simulink model "HVModAL_Fahrzeugmodell"  (R2015b)
settings: Solver=ode1  StartTime=0  StopTime=drp.driving_cycle.tstop  FixedStep=sim_params.Ts  RelTol=1e-5
PreLoadFcn:
  | % Add paths
  | addpath data
  | addpath(genpath('library'))
StartFcn:
  | Simulation.StartTime = tic;
StopFcn:
  | Simulation.DurationTime = toc(Simulation.StartTime);
undefined symbols (not defined in the file or in its folder): Batteries, BMS, BMS_Bat_, C_Nenn_DCDC1, C_Nenn_DCDC2, d2d, DC, DCDC_Converter_efficiency, DcDc_Converters, Dcl, drp, drv, elm, gen, gin, Hdc, hdc, HV, hvb, Hvb, ice, ldc, lib_dcl, lib_hdc, lib_hvb, lib_veh, Link, lossestable, mask_LUT_OCV, mask_LUT_OCV_SOC, mask_LUT_OCV_Temperature, mask_LUT_R, mask_LUT_Rs, mask_LUT_Rs_SOC, mask_LUT_Rs_Temperature, sim_params, speedvec, torquevec, tri, veh, Veh, Vehicle_Chassis
libraries: simulink x29, lib_tri_modules x7, lib_hdc_module x5, lib_gearbox x4, lib_hvb_battery_pack x3, cstblocks x3, PowerLimitBlock x2, MultiCellLibrary x2, lib_aux x1, lib_drv x1, lib_gen x1, lib_elm x1
(part 1 of 7)
settings Model: Creator=abu  LastModifiedBy=hangyang
settings SolverCC: AutoInsertRateTranBlk=on
settings DataIOCC: SaveFormat=Array  SignalLoggingSaveFormat=ModelDataLogs
settings OptimizationCC: DefaultParameterBehavior=Inlined
settings DebuggingCC: ReadBeforeWriteMsg=DisableAll  WriteAfterWriteMsg=DisableAll  WriteAfterReadMsg=DisableAll  CheckSSInitialOutputMsg=off  UnderspecifiedInitializationDetection=Classic  MergeDetectMultiDrivingBlocksExec=none  SolverPrmCheckMsg=warning  MultiTaskDSMMsg=none  MultiTaskCondExecSysMsg=none  UnconnectedInputMsg=none  UnconnectedOutputMsg=none  UnconnectedLineMsg=none  StateNameClashWarn=warning
settings HardwareCC: ProdBitPerPointer=32  ProdLargestAtomicFloat=None  ProdIntDivRoundTo=Undefined  ProdEndianess=Unspecified  ProdWordSize=32  ProdHWDeviceType=32-bit Generic
settings ModelReferenceCC: UpdateModelReferenceTargets=IfOutOfDate
settings SFSimCC: SFSimEcho=off
settings GRTTargetCC: GeneratePreprocessorConditionals=Disable all
settings ConfigComp: CovModelRefEnable=Off  CovSFcnEnable=off

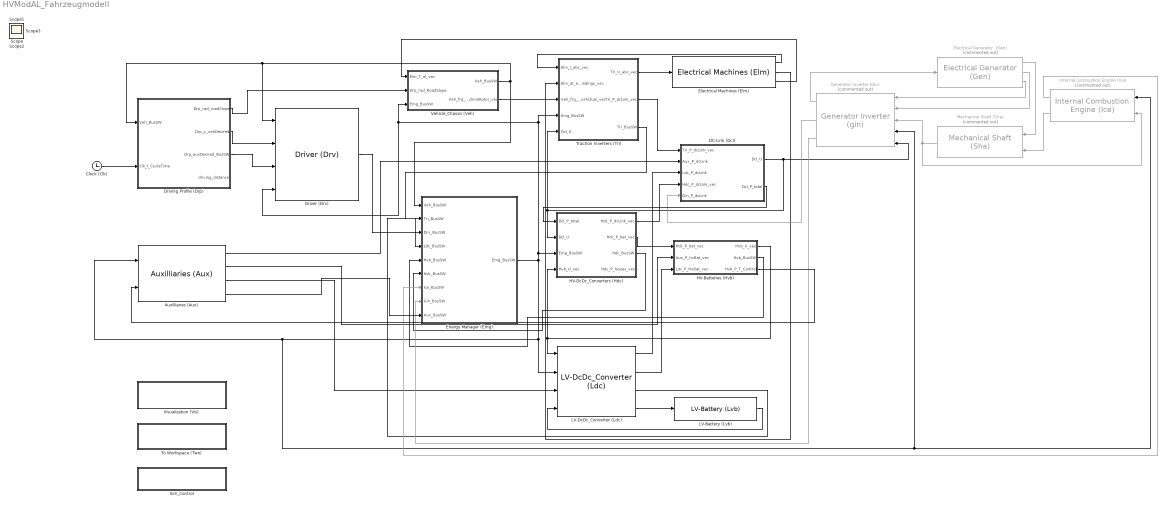
== system HVModAL_Fahrzeugmodell ==
  Auxilliaries (Aux) : lib_aux/Auxilliaries (Aux)
  Clock (Clk) : Clock
  DC-Link (Dcl) : Subsystem  AncestorBlock=lib_dcl/DC-Link (Dcl)
  Driver (Drv) : lib_drv/Driver (Drv)
  Driving Profile (Drp) : Subsystem  AncestorBlock=lib_drp/Driving Profile (Drp)
  Electrical Generator  (Gen) : lib_gen/Electrical Generator  (Gen)  Commented=on
  Electrical Machines (Elm) : lib_elm/Electrical Machines (Elm)
  Energy Manager (Emg) : Subsystem  AncestorBlock=lib_emg/Energy Manager (Emg)
  Generator Inverter (Gin) : lib_gin/Generator Inverter (gin)  Commented=on
  HV-Batteries (Hvb) : Subsystem  AncestorBlock=lib_hvb/HV-Batteries (Hvb)
  HV-DcDc_Converters (Hdc) : Subsystem  AncestorBlock=lib_hdc/HV-DcDc_Converters (Hdc)
  Internal Combustion Engine (Ice) : lib_ice/Internal Combustion Engine (Ice)  Commented=on
  LV-Battery (Lvb) : lib_lvb/LV-Battery (Lvb)
  LV-DcDc_Converter (Ldc) : lib_ldc/LV-DcDc_Converter (Ldc)
  Mechanical Shaft (Sha) : lib_Sha/Mechanical Shaft (Sha)  Commented=on
  Sim_Control : Subsystem
  To Workspace (Two) : Subsystem
  Traction Inverters (Tri) : Subsystem  AncestorBlock=lib_tri/Traction Inverters (Tri)
  Vehicle_Chassis (Veh) : Subsystem  AncestorBlock=lib_veh/Vehicle_Chassis (Veh)
  Visualization (Vis) : Subsystem
  Scope{,1..3} (4 alike) : Scope
  wires:
  Clock (Clk)/1 -> Driving Profile (Drp)/2(Clk_t_CycleTime)
  HV-Batteries (Hvb)/1(Hvb_U_vec) -> LV-DcDc_Converter (Ldc)/1, HV-DcDc_Converters (Hdc)/4(Hvb_U_vec)
  Vehicle_Chassis (Veh)/1(Veh_BusSW) -> Energy Manager (Emg)/1(Veh_BusSW), Driver (Drv)/1, Driving Profile (Drp)/1(Veh_BusSW)
  LV-DcDc_Converter (Ldc)/2 -> HV-Batteries (Hvb)/3(Ldc_P_HvBat_vec)
  Traction Inverters (Tri)/1(Tri_U_abc_vec) -> Electrical Machines (Elm)/1
  LV-DcDc_Converter (Ldc)/4 -> LV-Battery (Lvb)/1
  LV-Battery (Lvb)/1 -> LV-DcDc_Converter (Ldc)/4
  Driving Profile (Drp)/1(Drp_rad_roadSlope) -> Vehicle_Chassis (Veh)/2(Drp_rad_RoadSlope)
  Traction Inverters (Tri)/2(Tri_P_dcLink_vec) -> DC-Link (Dcl)/1(Tri_P_dcLink_vec)
  HV-DcDc_Converters (Hdc)/1(Hdc_P_dcLink_vec) -> DC-Link (Dcl)/4(Hdc_P_dcLink_vec)
  Auxilliaries (Aux)/3 -> LV-DcDc_Converter (Ldc)/3
  LV-DcDc_Converter (Ldc)/1 -> DC-Link (Dcl)/3(Ldc_P_dcLink)
  Energy Manager (Emg)/1(Emg_BusSW) -> Vehicle_Chassis (Veh)/3(Emg_BusSW), Driver (Drv)/4, Traction Inverters (Tri)/4(Emg_BusSW), HV-DcDc_Converters (Hdc)/3(Emg_BusSW), Internal Combustion Engine (Ice)/1, Generator Inverter (Gin)/4, Auxilliaries (Aux)/1, LV-DcDc_Converter (Ldc)/2
  DC-Link (Dcl)/1(Dcl_U) -> Traction Inverters (Tri)/5(Dcl_U), HV-DcDc_Converters (Hdc)/2(Dcl_U), Generator Inverter (Gin)/5
  Auxilliaries (Aux)/1 -> DC-Link (Dcl)/2(Aux_P_dcLink)
  HV-DcDc_Converters (Hdc)/2(Hdc_P_bat_vec) -> HV-Batteries (Hvb)/1(Hdc_P_bat_vec)
  Auxilliaries (Aux)/2 -> HV-Batteries (Hvb)/2(Aux_P_hvBat_vec)
  Vehicle_Chassis (Veh)/2(Veh_frq_machineRotor_vec) -> Traction Inverters (Tri)/3(Veh_frq_RotorActual_vec)
  Driver (Drv)/1 -> Energy Manager (Emg)/3("Drv_BusSW ")
  LV-DcDc_Converter (Ldc)/3 -> Energy Manager (Emg)/4(Ldc_BusSW)
  HV-DcDc_Converters (Hdc)/3(Hdc_BusSW) -> Energy Manager (Emg)/6(Hdc_BusSW)
  HV-Batteries (Hvb)/2(Hvb_BusSW) -> Energy Manager (Emg)/5(Hvb_BusSW)
  Traction Inverters (Tri)/3("Tri_BusSW ") -> Energy Manager (Emg)/2(Tri_BusSW)
  Electrical Machines (Elm)/1 -> Traction Inverters (Tri)/1(Elm_I_abc_vec)
  Electrical Machines (Elm)/2 -> Traction Inverters (Tri)/2(Elm_at_endWindings_vec)
  Generator Inverter (Gin)/2 -> DC-Link (Dcl)/5(Gin_P_dcLink)
  Generator Inverter (Gin)/1 -> Electrical Generator  (Gen)/1
  Electrical Generator  (Gen)/3 -> Generator Inverter (Gin)/1
  Electrical Generator  (Gen)/2 -> Generator Inverter (Gin)/2
  Mechanical Shaft (Sha)/1 -> Internal Combustion Engine (Ice)/2, Generator Inverter (Gin)/3
  Electrical Generator  (Gen)/1 -> Mechanical Shaft (Sha)/1
  Internal Combustion Engine (Ice)/2 -> Mechanical Shaft (Sha)/2
  Internal Combustion Engine (Ice)/1 -> Energy Manager (Emg)/7(Ice_BusSW)
  Generator Inverter (Gin)/3 -> Energy Manager (Emg)/8(Gin_BusSW)
  DC-Link (Dcl)/2(Dcl_P_total) -> HV-DcDc_Converters (Hdc)/1(Dcl_P_total)
  Electrical Machines (Elm)/3 -> Vehicle_Chassis (Veh)/1(Elm_T_el_vec)
  Driving Profile (Drp)/2(Drp_v_vehDesired) -> Driver (Drv)/2
  Driving Profile (Drp)/3(Drp_auxDesired_BusSW) -> Driver (Drv)/3
  Auxilliaries (Aux)/4 -> Energy Manager (Emg)/9("Aux_BusSW ")
  HV-Batteries (Hvb)/3(Hvb_P_T_Control) -> Auxilliaries (Aux)/2

== system HVModAL_Fahrzeugmodell/DC-Link (Dcl) ==
  note: edited by Jan: if this signal is cut, we don't have a direct algebraic loop
  Tri_P_dcLink_vec : Inport
  Aux_P_dcLink : Inport  Port=2
  Ldc_P_dcLink : Inport  Port=3
  Hdc_P_dcLink_vec : Inport  Port=4
  Gin_P_dcLink : Inport  Port=5
  Add : Sum  Inputs=+-
  Bus Creator : BusCreator  Inputs=4
  Dcl Voltage Calculation : Subsystem
  Delay : Delay  DelayLength=1  InitialCondition=0
  Gain : Gain  Gain=0
  Model Info : simulink/Model-Wide Utilities/Model Info  Frame=on  DisplayStringWithTags=|  HorizontalTextAlignment=Center  LeftAlignmentValue=0.5  SourceBlockDiagram=HVModAL_Fahrzeugmodell  TagMaxNumber=20
      | Responsibility
      | ISEA
      | 
      | Model Version: %<ModelVersion>
      | Last modified: %<LastModificationDate>
  Subtract1 : Sum  Inputs=+++++
  Sum of Elements : Sum  Inputs=+  SaturateOnIntegerOverflow=on
  Sum of Elements1 : Sum  Inputs=+  CollapseDim=2  SaturateOnIntegerOverflow=on
  Dcl_U : Outport
  Dcl_P_total : Outport  Port=2
  tag scope: Dcl_BusPB_toworkspace=global
  wires:
  Hdc_P_dcLink_vec/1 -> Sum of Elements/1
  Gin_P_dcLink/1 -> Gain/1
  Ldc_P_dcLink/1 -> Subtract1/4
  Sum of Elements/1 -> Delay/1
  Subtract1/1 -> Dcl Voltage Calculation/1(P), Bus Creator/3, Add/1  "Dcl_P_totalwoHdcPdcLink"
  Add/1 -> Dcl_P_total/1, Bus Creator/2  "Dcl_P_total"
  Aux_P_dcLink/1 -> Subtract1/3
  Gain/1 -> Subtract1/1
  Dcl Voltage Calculation/1(Dcl_U) -> Bus Creator/1, Dcl_U/1  "Dcl_U"
  Tri_P_dcLink_vec/1 -> Sum of Elements1/1
  Sum of Elements1/1 -> Subtract1/2
  Bus Creator/1 -> [Dcl_BusPB_toworkspace]
  Delay/1 -> Bus Creator/4  "Hdc_P_dcLink"

== system HVModAL_Fahrzeugmodell/Driving Profile (Drp) ==
  Veh_BusSW : Inport
  Clk_t_CycleTime : Inport  Port=2
  Bus Creator : BusCreator  Inputs=4
  Bus Creator1 : BusCreator  Inputs=3
  Load{1..4} (4 alike) : Constant  Value=0
  Model Info : simulink/Model-Wide Utilities/Model Info  Frame=on  DisplayStringWithTags=|  HorizontalTextAlignment=Center  LeftAlignmentValue=0.5  SourceBlockDiagram=HVModAL_Fahrzeugmodell  TagMaxNumber=20
      | Responsibility
      | ISEA
      | 
      | Model Version: %<ModelVersion>
      | Last modified: %<LastModificationDate>
  Slope Lookup : Lookup_n-D  NumberOfTableDimensions=1  BreakpointsForDimension1=drp.driving_cycle.slope(:,1)  Table=drp.driving_cycle.slope(:,2)  InternalRulePriority=Speed  RndMeth=Simplest  InputSameDT=on
  Speed Lookup : Lookup_n-D  NumberOfTableDimensions=1  BreakpointsForDimension1=drp.driving_cycle.speed(:,1)  Table=drp.driving_cycle.speed(:,2)  InternalRulePriority=Speed  RndMeth=Simplest  InputSameDT=on
  Terminator : Terminator
  drp_driving_distance[Km] : Constant  Value=500
  "km/h -> m/s" : Gain  Gain=1/3.6
  Drp_rad_roadSlope : Outport
  Drp_v_vehDesired : Outport  Port=2
  Drp_auxDesired_BusSW : Outport  Port=3
  "driving_distance " : Outport  Port=4
  tag scope: Drp_SWBus_toworkspace=global
  wires:
  "km/h -> m/s"/1 -> Bus Creator1/1, Drp_v_vehDesired/1  "Drp_v_vehDesired"
  Veh_BusSW/1 -> Terminator/1
  Clk_t_CycleTime/1 -> Slope Lookup/1, Speed Lookup/1
  Slope Lookup/1 -> Bus Creator1/2, Drp_rad_roadSlope/1  "Drp_rad_roadSlope"
  Bus Creator/1 -> Bus Creator1/3, Drp_auxDesired_BusSW/1  "Drp_auxDesired_BusSW"
  Load4/1 -> Bus Creator/4
  Load3/1 -> Bus Creator/3
  Load2/1 -> Bus Creator/2
  Load1/1 -> Bus Creator/1
  Bus Creator1/1 -> [Drp_SWBus_toworkspace]
  Speed Lookup/1 -> "km/h -> m/s"/1
  drp_driving_distance[Km]/1 -> "driving_distance "/1

== system HVModAL_Fahrzeugmodell/Energy Manager (Emg) ==
  note: Emg_battery_control_case
  note: Attention: SOC equalization strategy forced (27.9.16, JaB)
  Veh_BusSW : Inport
  Tri_BusSW : Inport  Port=2
  "Drv_BusSW " : Inport  Port=3
  Ldc_BusSW : Inport  Port=4
  Hvb_BusSW : Inport  Port=5
  Hdc_BusSW : Inport  Port=6
  Ice_BusSW : Inport  Port=7
  Gin_BusSW : Inport  Port=8
  "Aux_BusSW " : Inport  Port=9
  Aux Control : Subsystem
  Battery Control : Subsystem
  Battery Control1 : Subsystem  Commented=through
      mask help: Simulink:masks:GenSFuncDesc_MD
      mask Help: eval('feval(''rtwprivate'',''rtwhelpview'',''rtw_sfcn_block'')');
  Bus Creator : BusCreator  Inputs=13
  Emg_P_lvDemand : Constant  Value=0
  Emg_P_lvDemand1 : Constant  Value=0
  Emg_U_dcLinkDemand : Constant  Value=veh.topology.Dcl_U
  Model Info : simulink/Model-Wide Utilities/Model Info  Frame=on  DisplayStringWithTags=|  HorizontalTextAlignment=Center  LeftAlignmentValue=0.5  SourceBlockDiagram=HVModAL_Fahrzeugmodell  TagMaxNumber=20
      | Responsibility
      | ISEA
      | 
      | Model Version: %<ModelVersion>
      | Last modified: %<LastModificationDate>
  Mux : Mux  Inputs=3
  Range Extender Control : Subsystem
  Terminator2 : Terminator
  "Torque Control motor (1 elm, 1 tri, 2 hdc, 2 bat)" : Torque_Control/Torque Control motor (1 elm, 1 tri, 2 hdc, 2 bat)
  at_Ambient : Constant  Value=25
  Emg_BusSW : Outport
  tag scope: EMG_BusSW_ToLogging=global, EMG_BusSW_ToWorkspace=global
  wires:
  Emg_P_lvDemand/1 -> Mux/3  "Emg_P_lvDemand"
  Emg_U_dcLinkDemand/1 -> Bus Creator/6  "Emg_U_dcLinkDemand"
  Bus Creator/1 -> Emg_BusSW/1, [EMG_BusSW_ToWorkspace], [EMG_BusSW_ToLogging]
  Tri_BusSW/1 -> "Torque Control motor (1 elm, 1 tri, 2 hdc, 2 bat)"/5, Aux Control/4(Tri_BusSW), Battery Control/3(Tri_BusSW)
  Ldc_BusSW/1 -> Terminator2/1
  Hdc_BusSW/1 -> "Torque Control motor (1 elm, 1 tri, 2 hdc, 2 bat)"/4
  Ice_BusSW/1 -> Range Extender Control/1(Ice_BusSW)
  Gin_BusSW/1 -> Range Extender Control/2(Gin_BusSW)
  Hvb_BusSW/1 -> Battery Control/1(Hvb_BusSW), "Torque Control motor (1 elm, 1 tri, 2 hdc, 2 bat)"/6
  Range Extender Control/1(Emg_fac_GenDeman) -> Bus Creator/9  "Emg_fac_GenDeman"
  "Torque Control motor (1 elm, 1 tri, 2 hdc, 2 bat)"/1 -> Bus Creator/1  "Emg_T_elDemand_vec"
  "Drv_BusSW "/1 -> "Torque Control motor (1 elm, 1 tri, 2 hdc, 2 bat)"/2
  "Torque Control motor (1 elm, 1 tri, 2 hdc, 2 bat)"/2 -> Bus Creator/2  "Emg_T_mechDemand"
  Battery Control/1(Emg_fac_powerDistribution_vec) -> Bus Creator/5  "Emg_fac_powerDistribution_vec"
  Aux Control/1(Emg_auxControl_BusSW) -> Bus Creator/8
  Veh_BusSW/1 -> Battery Control/2(Veh_BusSW), "Torque Control motor (1 elm, 1 tri, 2 hdc, 2 bat)"/3
  Mux/1 -> Bus Creator/7  "Emg_P_lvdemand"
  Emg_P_lvDemand1/1 -> Mux/2, Mux/1
  at_Ambient/1 -> Bus Creator/10  "Emg_at_Ambient"
  "Torque Control motor (1 elm, 1 tri, 2 hdc, 2 bat)"/3 -> Bus Creator/3  "Emg_Degradation_vec"
  [Tri_BusPB_toWorkspace] -> Aux Control/1(Tri_BusPW)
  [Hdc_PBBus_toWorkspace] -> Aux Control/2(Hdc_BusPW)
  [Hvb_PBbus_toworkspace] -> Aux Control/3(Hvb_BusPW)
  "Torque Control motor (1 elm, 1 tri, 2 hdc, 2 bat)"/4 -> Bus Creator/4  "Emg_Degradation_vec_driver"
  "Aux_BusSW "/1 -> Battery Control/4("Aux_BusSW "), "Torque Control motor (1 elm, 1 tri, 2 hdc, 2 bat)"/1
  "Torque Control motor (1 elm, 1 tri, 2 hdc, 2 bat)"/5 -> Bus Creator/11  "Emg_Gearbox_vec"
  Battery Control/2(case) -> Bus Creator/12
  Battery Control/3(I_rex) -> Bus Creator/13

== system HVModAL_Fahrzeugmodell/HV-Batteries (Hvb) ==
  note: inserted to break algebraic loop
  note: power vector demanded by
      | DC/DC converters
  note: power vector demanded by
      | Auxiliaries
  note: power vector demanded by
      | low voltage DC/DC conv.
  Hdc_P_bat_vec : Inport
  Aux_P_hvBat_vec : Inport  Port=2
  Ldc_P_HvBat_vec : Inport  Port=3
  Add : Sum  Inputs=+++++
  Bat_1 : Subsystem  AncestorBlock=lib_hvb_battery_pack/Bat_1  mask{mask_Num_Temp_Sensoren=hvb.Bat1.Num_Temp_Sensors, mask_Num_Zellen_el_par=hvb.Bat1.Num_Cells_el_par, mask_Num_Zellen_el_ser=hvb.Bat1.Num_Cells_el_ser, mask_init_SOC=hvb.Bat1.SOC_init, mask_U_Nenn=hvb.Bat1.cell.V_nom, mask_config_str=hvb.Bat1.cell.CONFIG_STR, mask_n_BatteryType=hvb.Bat1.cell.type, mask_b_Bat_Avail=hvb.Bat1.phys_avail, mask_f_C_nom=hvb.Bat1.cell.C_nom, mask_I_max_cha=hvb.Bat1.cell.I_max_cha, mask_I_max_disch=hvb.Bat1.cell.I_max_disch, mask_m_battery_pack=hvb.Bat1.pack_mass.sum, mask_P_max_disch=hvb.Bat1.P_max_disch, mask_m_cell=hvb.Bat1.cell.m_cell, mask_thickness_cell=hvb.Bat1.cell.thickness_cell, mask_width_cell=hvb.Bat1.cell.width_cell, mask_cooling_method=hvb.Bat1.cooling_system, mask_height_cell=hvb.Bat1.cell.height_cell, mask_volume_cell=hvb.Bat1.cell.volume_cell, mask_v_Radial_Fan=10, mask_sum_packvolume=hvb.Bat1.pack_volume.sum, mask_cooling_area=hvb.Bat1.cooling_area, mask_housing_width=hvb.Bat1.pack_volume.width, mask_housing_height=hvb.Bat1.pack_volume.heigth, mask_housing_length=hvb.Bat1.pack_volume.length}
      mask prompts: mask_Num_Temp_Sensoren "Number of temperature sensors"; mask_Num_Zellen_el_par "Number of cells in parallel"; mask_Num_Zellen_el_ser "Number of cells in series"; mask_init_SOC "Initial SOC [%]"; mask_U_Nenn "Cell nominal voltage [V]"; mask_config_str "Battery pack parameter"; mask_n_BatteryType "Battery Type"; mask_b_Bat_Avail "Battery Available"; mask_f_C_nom "Cell nominal Capacity"; mask_I_max_cha "I max charge cell in A"; mask_I_max_disch "I max discharge cell in A"; mask_m_battery_pack "battery pack mass"; mask_P_max_disch "P max discharge"; mask_m_cell "Cell mass"; mask_thickness_cell "Cell Thickness"; mask_width_cell "Cell Width"; mask_cooling_method "Cooling"; mask_height_cell "Cell Height"; mask_volume_cell "Cell Volume"; mask_v_Radial_Fan "v Radial Fan"; mask_sum_packvolume "Volume Sum Pack"; mask_cooling_area "Cooling Area"; mask_housing_width "Housing Width"; mask_housing_height "Housing Height"; mask_housing_length "Housing Length"
  Bat_2 : Subsystem  AncestorBlock=lib_hvb_battery_pack/Bat_1  mask{mask_Num_Temp_Sensoren=hvb.Bat2.Num_Temp_Sensors, mask_Num_Zellen_el_par=hvb.Bat2.Num_Cells_el_par, mask_Num_Zellen_el_ser=hvb.Bat2.Num_Cells_el_ser, mask_init_SOC=hvb.Bat2.SOC_init, mask_U_Nenn=hvb.Bat2.cell.V_nom, mask_config_str=hvb.Bat2.cell.CONFIG_STR, mask_n_BatteryType=hvb.Bat2.cell.type, mask_b_Bat_Avail=hvb.Bat2.phys_avail, mask_f_C_nom=hvb.Bat2.cell.C_nom, mask_I_max_cha=hvb.Bat2.cell.I_max_cha, mask_I_max_disch=hvb.Bat2.cell.I_max_disch, mask_m_battery_pack=hvb.Bat2.pack_mass.sum, mask_P_max_disch=hvb.Bat2.P_max_disch, mask_m_cell=hvb.Bat2.cell.m_cell, mask_thickness_cell=hvb.Bat2.cell.thickness_cell, mask_width_cell=hvb.Bat2.cell.width_cell, mask_cooling_method=hvb.Bat2.cooling_system, mask_height_cell=hvb.Bat2.cell.height_cell, mask_volume_cell=hvb.Bat2.cell.volume_cell, mask_v_Radial_Fan=10, mask_sum_packvolume=hvb.Bat2.pack_volume.sum, mask_cooling_area=hvb.Bat2.cooling_area, mask_housing_width=hvb.Bat2.pack_volume.width, mask_housing_height=hvb.Bat2.pack_volume.heigth, mask_housing_length=hvb.Bat2.pack_volume.length}
      mask prompts: mask_Num_Temp_Sensoren "Number of temperature sensors"; mask_Num_Zellen_el_par "Number of cells in parallel"; mask_Num_Zellen_el_ser "Number of cells in series"; mask_init_SOC "Initial SOC [%]"; mask_U_Nenn "Cell nominal voltage [V]"; mask_config_str "Battery pack parameter"; mask_n_BatteryType "Battery Type"; mask_b_Bat_Avail "Battery Available"; mask_f_C_nom "Cell nominal Capacity"; mask_I_max_cha "I max charge cell in A"; mask_I_max_disch "I max discharge cell in A"; mask_m_battery_pack "battery pack mass"; mask_P_max_disch "P max discharge"; mask_m_cell "Cell mass"; mask_thickness_cell "Cell Thickness"; mask_width_cell "Cell Width"; mask_cooling_method "Cooling"; mask_height_cell "Cell Height"; mask_volume_cell "Cell Volume"; mask_v_Radial_Fan "v Radial Fan"; mask_sum_packvolume "Volume Sum Pack"; mask_cooling_area "Cooling Area"; mask_housing_width "Housing Width"; mask_housing_height "Housing Height"; mask_housing_length "Housing Length"
  Bat_3 : lib_hvb_battery_pack/Bat_1  mask_Num_Temp_Sensoren=hvb.Bat3.Num_Temp_Sensors  mask_Num_Zellen_el_par=hvb.Bat3.Num_Cells_el_par  mask_Num_Zellen_el_ser=hvb.Bat3.Num_Cells_el_ser  mask_init_SOC=hvb.Bat3.SOC_init  mask_U_Nenn=hvb.Bat3.cell.V_nom  mask_config_str=hvb.Bat3.cell.CONFIG_STR  mask_n_BatteryType=hvb.Bat3.cell.type  mask_b_Bat_Avail=hvb.Bat3.phys_avail  mask_f_C_nom=hvb.Bat3.cell.C_nom  mask_I_max_cha=hvb.Bat3.cell.I_max_cha  mask_I_max_disch=hvb.Bat3.cell.I_max_disch  mask_m_battery_pack=hvb.Bat3.pack_mass.sum  mask_P_max_disch=hvb.Bat3.P_max_disch  mask_m_cell=hvb.Bat3.cell.m_cell  mask_thickness_cell=hvb.Bat3.cell.thickness_cell  mask_width_cell=hvb.Bat3.cell.width_cell  mask_cooling_method=hvb.Bat3.cooling_system  mask_height_cell=hvb.Bat3.cell.height_cell  mask_volume_cell=hvb.Bat3.cell.volume_cell  mask_v_Radial_Fan=10  mask_sum_packvolume=hvb.Bat3.pack_volume.sum  mask_cooling_area=hvb.Bat3.cooling_area  mask_housing_width=hvb.Bat3.pack_volume.width  mask_housing_height=hvb.Bat3.pack_volume.heigth  mask_housing_length=hvb.Bat3.pack_volume.length
  Bat_4 : lib_hvb_battery_pack/Bat_1  mask_Num_Temp_Sensoren=hvb.Bat4.Num_Temp_Sensors  mask_Num_Zellen_el_par=hvb.Bat4.Num_Cells_el_par  mask_Num_Zellen_el_ser=hvb.Bat4.Num_Cells_el_ser  mask_init_SOC=hvb.Bat4.SOC_init  mask_U_Nenn=hvb.Bat4.cell.V_nom  mask_config_str=hvb.Bat4.cell.CONFIG_STR  mask_n_BatteryType=hvb.Bat4.cell.type  mask_b_Bat_Avail=hvb.Bat4.phys_avail  mask_f_C_nom=hvb.Bat4.cell.C_nom  mask_I_max_cha=hvb.Bat4.cell.I_max_cha  mask_I_max_disch=hvb.Bat4.cell.I_max_disch  mask_m_battery_pack=hvb.Bat4.pack_mass.sum  mask_P_max_disch=hvb.Bat4.P_max_disch  mask_m_cell=hvb.Bat4.cell.m_cell  mask_thickness_cell=hvb.Bat4.cell.thickness_cell  mask_width_cell=hvb.Bat4.cell.width_cell  mask_cooling_method=hvb.Bat4.cooling_system  mask_height_cell=hvb.Bat4.cell.height_cell  mask_volume_cell=hvb.Bat4.cell.volume_cell  mask_v_Radial_Fan=10  mask_sum_packvolume=hvb.Bat4.pack_volume.sum  mask_cooling_area=hvb.Bat4.cooling_area  mask_housing_width=hvb.Bat4.pack_volume.width  mask_housing_height=hvb.Bat4.pack_volume.heigth  mask_housing_length=hvb.Bat4.pack_volume.length
  Bat_5 : lib_hvb_battery_pack/Bat_1  mask_Num_Temp_Sensoren=hvb.Bat5.Num_Temp_Sensors  mask_Num_Zellen_el_par=hvb.Bat5.Num_Cells_el_par  mask_Num_Zellen_el_ser=hvb.Bat5.Num_Cells_el_ser  mask_init_SOC=hvb.Bat5.SOC_init  mask_U_Nenn=hvb.Bat5.cell.V_nom  mask_config_str=hvb.Bat5.cell.CONFIG_STR  mask_n_BatteryType=hvb.Bat5.cell.type  mask_b_Bat_Avail=hvb.Bat5.phys_avail  mask_f_C_nom=hvb.Bat5.cell.C_nom  mask_I_max_cha=hvb.Bat5.cell.I_max_cha  mask_I_max_disch=hvb.Bat5.cell.I_max_disch  mask_m_battery_pack=hvb.Bat5.pack_mass.sum  mask_P_max_disch=hvb.Bat5.P_max_disch  mask_m_cell=hvb.Bat5.cell.m_cell  mask_thickness_cell=hvb.Bat5.cell.thickness_cell  mask_width_cell=hvb.Bat5.cell.width_cell  mask_cooling_method=hvb.Bat5.cooling_system  mask_height_cell=hvb.Bat5.cell.height_cell  mask_volume_cell=hvb.Bat5.cell.volume_cell  mask_v_Radial_Fan=10  mask_sum_packvolume=hvb.Bat5.pack_volume.sum  mask_cooling_area=hvb.Bat5.cooling_area  mask_housing_width=hvb.Bat5.pack_volume.width  mask_housing_height=hvb.Bat5.pack_volume.heigth  mask_housing_length=hvb.Bat5.pack_volume.length
  Bus Creator : BusCreator  Inputs=5
  Bus Creator1 : BusCreator  Inputs=5
  Bus Selector{,1..3,5} (5 alike) : BusSelector  OutputSignals=Total_Voltage_V
  Bus Selector4 : BusSelector  OutputSignals=PB_Bat1,PB_Bat2,PB_Bat3,PB_Bat4,PB_Bat5
  Bus Selector6 : BusSelector  OutputSignals=PB_Bat1.P_T_control_power_W,PB_Bat2.P_T_control_power_W,PB_Bat3.P_T_control_power_W,PB_Bat4.P_T_control_power_W,PB_Bat5.P_T_control_power_W
  Constant : Constant  Value=hvb.Bat1.phys_avail
  Constant1 : Constant  Value=hvb.Bat5.phys_avail
  Constant2 : Constant  Value=hvb.Bat2.phys_avail
  Constant3 : Constant  Value=hvb.Bat3.phys_avail
  Constant4 : Constant  Value=hvb.Bat4.phys_avail
  Delay : Delay  DelayLength=1  InitialCondition=0
  Delay1 : Delay  DelayLength=1  InitialCondition=0
  Demux : Demux  Outputs=5
  Model Info : simulink/Model-Wide Utilities/Model Info  Frame=on  DisplayStringWithTags=|  HorizontalTextAlignment=Center  LeftAlignmentValue=0.5  SourceBlockDiagram=HVModAL_Fahrzeugmodell  TagMaxNumber=20
      | Last modified
      | %<LastModificationDate>
      | 
      | Model Version
      | %<ModelVersion>
      | 
      | responsible: ISEA-ESS
  Mux : Mux  Inputs=5
  Scope : Scope
  Sum : Sum  Inputs=+++
  T_ambient : Constant  Value=hvb.Bat1.T_ambient
  Hvb_U_vec : Outport
  Hvb_BusSW : Outport  Port=2
  Hvb_P_T_Control : Outport  Port=3
  tag scope: Hvb_PBbus_toworkspace=global, Hvb_SWbus_toworkspace=global
  wires:
  Ldc_P_HvBat_vec/1 -> Sum/3
  Hdc_P_bat_vec/1 -> Sum/1
  Aux_P_hvBat_vec/1 -> Sum/2
  Bus Creator/1 -> Delay/1
  Demux/2 -> Bat_2/1(P_Bat_W), Scope/1
  Demux/1 -> Bat_1/1(P_Bat_W)
  Demux/3 -> Bat_3/1
  Mux/1 -> Hvb_U_vec/1
  Demux/4 -> Bat_4/1
  Demux/5 -> Bat_5/1
  Bat_1/1(PB_Bat) -> Bus Creator1/1  "PB_Bat1"
  Bat_2/1(PB_Bat) -> Bus Creator1/2  "PB_Bat2"
  Bat_3/1 -> Bus Creator1/3  "PB_Bat3"
  Bat_4/1 -> Bus Creator1/4  "PB_Bat4"
  Bat_5/1 -> Bus Creator1/5  "PB_Bat5"
  Bus Selector2/1 -> Mux/3  "<Total_Voltage_V>"
  Bus Selector5/1 -> Mux/5  "<Total_Voltage_V>"
  Bus Selector3/1 -> Mux/4  "<Total_Voltage_V>"
  Bus Selector/1 -> Mux/1  "<Total_Voltage_V>"
  Bus Selector1/1 -> Mux/2  "<Total_Voltage_V>"
  Bus Creator1/1 -> Bus Selector6/1, [Hvb_PBbus_toworkspace], Bus Selector4/1
  Bus Selector4/1 -> Bus Selector/1  "<PB_Bat1>"
  Bus Selector4/2 -> Bus Selector1/1  "<PB_Bat2>"
  Bus Selector4/3 -> Bus Selector2/1  "<PB_Bat3>"
  Bus Selector4/4 -> Bus Selector3/1  "<PB_Bat4>"
  Bus Selector4/5 -> Bus Selector5/1  "<PB_Bat5>"
  Bat_1/2(SB_Bat) -> Bus Creator/1  "SB_Bat1"
  Bat_2/2(SB_Bat) -> Bus Creator/2  "SB_Bat2"
  Bat_3/2 -> Bus Creator/3  "SB_Bat3"
  Bat_4/2 -> Bus Creator/4  "SB_Bat4"
  Bat_5/2 -> Bus Creator/5  "SB_Bat5"
  Sum/1 -> Demux/1
  Constant2/1 -> Bat_2/Enable
  Constant3/1 -> Bat_3/Enable
  Constant4/1 -> Bat_4/Enable
  Constant1/1 -> Bat_5/Enable
  Delay/1 -> [Hvb_SWbus_toworkspace], Hvb_BusSW/1
  T_ambient/1 -> Bat_1/2(T_ambient), Bat_5/2, Bat_4/2, Bat_3/2, Bat_2/2(T_ambient)
  Constant/1 -> Bat_1/Enable
  Bus Selector6/3 -> Add/3  "<P_T_control_power_W>"
  Bus Selector6/2 -> Add/2  "<P_T_control_power_W>"
  Bus Selector6/4 -> Add/4  "<P_T_control_power_W>"
  Bus Selector6/1 -> Add/1  "<P_T_control_power_W>"
  Bus Selector6/5 -> Add/5  "<P_T_control_power_W>"
  Add/1 -> Delay1/1
  Delay1/1 -> Hvb_P_T_Control/1

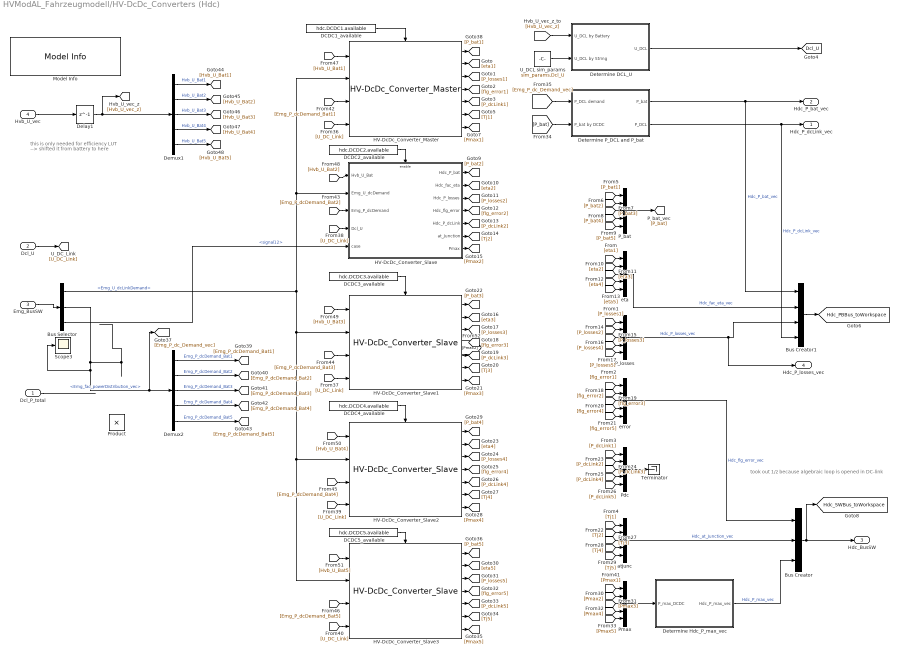
== system HVModAL_Fahrzeugmodell/HV-DcDc_Converters (Hdc) ==
  note: this is only needed for efficiency LUT
      | --> shifted it from battery to here
  note: took out 1/z because algebraic loop is opened in DC-link
  Dcl_P_total : Inport
  Dcl_U : Inport  Port=2
  Emg_BusSW : Inport  Port=3
  Hvb_U_vec : Inport  Port=4
  Bus Creator : BusCreator  Inputs=3
  Bus Creator1 : BusCreator  Inputs=4
  Bus Selector : BusSelector  OutputSignals=Emg_U_dcLinkDemand,Emg_fac_powerDistribution_vec,signal12
  DCDC1_available : Constant  Value=hdc.DCDC1.available
  DCDC2_available : Constant  Value=hdc.DCDC2.available
  DCDC3_available : Constant  Value=hdc.DCDC3.available
  DCDC4_available : Constant  Value=hdc.DCDC4.available
  DCDC5_available : Constant  Value=hdc.DCDC5.available
  Delay1 : Delay  DelayLength=1  InitialCondition=0
  Demux1 : Demux  Outputs=5
  Demux2 : Demux  Outputs=5
  Determine DCL_U : Subsystem
  Determine Hdc_P_max_vec : Subsystem
  Determine P_DCL and P_bat : Subsystem
  HV-DcDc_Converter_Master : lib_hdc_module/HV-DcDc_Converter_Master  DCDCname=hdc.DCDC1
  HV-DcDc_Converter_Slave : Subsystem  AncestorBlock=lib_hdc_module/HV-DcDc_Converter_Slave  mask{DCDCname=hdc.DCDC2}
      mask prompts: DCDCname "DCDC Struct"
  HV-DcDc_Converter_Slave1 : lib_hdc_module/HV-DcDc_Converter_Slave  DCDCname=hdc.DCDC2
  HV-DcDc_Converter_Slave2 : lib_hdc_module/HV-DcDc_Converter_Slave  DCDCname=hdc.DCDC2
  HV-DcDc_Converter_Slave3 : lib_hdc_module/HV-DcDc_Converter_Slave  DCDCname=hdc.DCDC2
  Model Info : simulink/Model-Wide Utilities/Model Info  Frame=on  DisplayStringWithTags=|  HorizontalTextAlignment=Center  LeftAlignmentValue=0.5  SourceBlockDiagram=HVModAL_Fahrzeugmodell  TagMaxNumber=20
      | Responsibility
      | ISEA
      | 
      | Model Version: %<ModelVersion>
      | Last modified: %<LastModificationDate>
  P_bat : Mux  Inputs=5
  P_losses : Mux  Inputs=5
  Pdc : Mux  Inputs=5
  Pmax : Mux  Inputs=5
  Product : Product
  Scope3 : Scope
  Terminator : Terminator
  U_DCL sim_params : Constant  Value=sim_params.Dcl_U
  atJunc : Mux  Inputs=5
  error : Mux  Inputs=5
  eta : Mux  Inputs=5
  Hdc_P_dcLink_vec : Outport
  Hdc_P_bat_vec : Outport  Port=2
  Hdc_BusSW : Outport  Port=3
  Hdc_P_losses_vec : Outport  Port=4
  tag scope: Dcl_U=global, Hdc_PBBus_toWorkspace=global, Hdc_SWBus_toWorkspace=global
  wires:
  [Tj5] -> atJunc/5
  [Tj2] -> atJunc/2
  [Tj3] -> atJunc/3
  [Tj4] -> atJunc/4
  [P_dcLink4] -> Pdc/4
  [P_dcLink5] -> Pdc/5
  [P_dcLink2] -> Pdc/2
  [P_dcLink3] -> Pdc/3
  [P_dcLink1] -> Pdc/1
  [flg_error3] -> error/3
  [flg_error5] -> error/5
  [flg_error4] -> error/4
  [flg_error2] -> error/2
  [P_losses4] -> P_losses/4
  [P_losses3] -> P_losses/3
  [P_losses2] -> P_losses/2
  [P_losses5] -> P_losses/5
  [eta5] -> eta/5
  [eta4] -> eta/4
  [eta3] -> eta/3
  [eta2] -> eta/2
  [P_bat5] -> P_bat/5
  [P_bat4] -> P_bat/4
  [P_bat3] -> P_bat/3
  HV-DcDc_Converter_Slave3/7 -> [Pmax5]
  HV-DcDc_Converter_Slave3/6 -> [Tj5]
  HV-DcDc_Converter_Slave3/5 -> [P_dcLink5]
  HV-DcDc_Converter_Slave3/4 -> [flg_error5]
  HV-DcDc_Converter_Slave3/3 -> [P_losses5]
  HV-DcDc_Converter_Slave3/2 -> [eta5]
  HV-DcDc_Converter_Slave3/1 -> [P_bat5]
  HV-DcDc_Converter_Slave2/7 -> [Pmax4]
  HV-DcDc_Converter_Slave2/6 -> [Tj4]
  HV-DcDc_Converter_Slave2/5 -> [P_dcLink4]
  HV-DcDc_Converter_Slave2/4 -> [flg_error4]
  HV-DcDc_Converter_Slave2/3 -> [P_losses4]
  HV-DcDc_Converter_Slave2/2 -> [eta4]
  HV-DcDc_Converter_Slave2/1 -> [P_bat4]
  HV-DcDc_Converter_Slave1/7 -> [Pmax3]
  HV-DcDc_Converter_Slave1/6 -> [Tj3]
  HV-DcDc_Converter_Slave1/5 -> [P_dcLink3]
  HV-DcDc_Converter_Slave1/4 -> [flg_error3]
  HV-DcDc_Converter_Slave1/3 -> [P_losses3]
  HV-DcDc_Converter_Slave1/2 -> [eta3]
  HV-DcDc_Converter_Slave1/1 -> [P_bat3]
  HV-DcDc_Converter_Slave/7(Pmax) -> [Pmax2]
  HV-DcDc_Converter_Slave/6(at_Junction) -> [Tj2]
  HV-DcDc_Converter_Slave/5(Hdc_P_dcLink) -> [P_dcLink2]
  HV-DcDc_Converter_Slave/4(Hdc_flg_error) -> [flg_error2]
  HV-DcDc_Converter_Slave/3(Hdc_P_losses) -> [P_losses2]
  HV-DcDc_Converter_Slave/2(Hdc_fac_eta) -> [eta2]
  [P_bat2] -> P_bat/2
  HV-DcDc_Converter_Slave/1(Hdc_P_bat) -> [P_bat2]
  HV-DcDc_Converter_Master/7 -> [Pmax1]
  HV-DcDc_Converter_Master/6 -> [Tj1]
  HV-DcDc_Converter_Master/5 -> [P_dcLink1]
  [flg_error1] -> error/1
  HV-DcDc_Converter_Master/4 -> [flg_error1]
  [P_losses1] -> P_losses/1
  [eta1] -> eta/1
  HV-DcDc_Converter_Master/3 -> [P_losses1]
  HV-DcDc_Converter_Master/2 -> [eta1]
  Demux2/5 -> [Emg_P_dcDemand_Bat5]  "Emg_P_dcDemand_Bat5"
  Demux2/4 -> [Emg_P_dcDemand_Bat4]  "Emg_P_dcDemand_Bat4"
  Demux2/3 -> [Emg_P_dcDemand_Bat3]  "Emg_P_dcDemand_Bat3"
  Emg_BusSW/1 -> Bus Selector/1
  Bus Creator/1 -> [Hdc_SWBus_toWorkspace], Hdc_BusSW/1
  Demux2/1 -> [Emg_P_dcDemand_Bat1]  "Emg_P_dcDemand_Bat1"
  P_losses/1 -> Hdc_P_losses_vec/1, Bus Creator1/3  "Hdc_P_losses_vec"
  P_bat/1 -> [P_bat]
  eta/1 -> Bus Creator1/2  "Hdc_fac_eta_vec"
  Bus Selector/1 -> HV-DcDc_Converter_Master/2, HV-DcDc_Converter_Slave/2(Emg_U_dcDemand), HV-DcDc_Converter_Slave1/2, HV-DcDc_Converter_Slave2/2, HV-DcDc_Converter_Slave3/2  "<Emg_U_dcLinkDemand>"
  Demux1/1 -> [Hvb_U_Bat1]  "Hvb_U_Bat1"
  Bus Selector/2 -> Demux2/1, [Emg_P_dc_Demand_vec], Scope3/1  "<Emg_fac_powerDistribution_vec>"
  Hvb_U_vec/1 -> Delay1/1
  DCDC2_available/1 -> HV-DcDc_Converter_Slave/Enable
  DCDC3_available/1 -> HV-DcDc_Converter_Slave1/Enable
  Demux1/2 -> [Hvb_U_Bat2]  "Hvb_U_Bat2"
  Demux1/5 -> [Hvb_U_Bat5]  "Hvb_U_Bat5"
  Demux1/4 -> [Hvb_U_Bat4]  "Hvb_U_Bat4"
  Demux1/3 -> [Hvb_U_Bat3]  "Hvb_U_Bat3"
  DCDC5_available/1 -> HV-DcDc_Converter_Slave3/Enable
  DCDC4_available/1 -> HV-DcDc_Converter_Slave2/Enable
  error/1 -> Bus Creator/1  "Hdc_flg_error_vec"
  atJunc/1 -> Bus Creator/2  "Hdc_at_Junction_vec"
  Pmax/1 -> Determine Hdc_P_max_vec/1(P_max_DCDC)
  DCDC1_available/1 -> HV-DcDc_Converter_Master/Enable
  Bus Creator1/1 -> [Hdc_PBBus_toWorkspace]
  Delay1/1 -> Demux1/1, [Hvb_U_vec_z]
  [Tj1] -> atJunc/1
  U_DCL sim_params/1 -> Determine DCL_U/2(U_DCL by String)
  Determine DCL_U/1(U_DCL) -> [Dcl_U]
  [Hvb_U_vec_z] -> Determine DCL_U/1(U_DCL by Battery)
  [P_bat] -> Determine P_DCL and P_bat/2(P_bat by DCDC)
  [Emg_P_dc_Demand_vec] -> Determine P_DCL and P_bat/1(P_DCL demand)
  Demux2/2 -> [Emg_P_dcDemand_Bat2]  "Emg_P_dcDemand_Bat2"
  Determine P_DCL and P_bat/1(P_bat) -> Bus Creator1/1, Hdc_P_bat_vec/1  "Hdc_P_bat_vec"
  Determine P_DCL and P_bat/2(P_DCL) -> Hdc_P_dcLink_vec/1, Bus Creator1/4  "Hdc_P_dcLink_vec"
  [U_DC_Link] -> HV-DcDc_Converter_Slave2/4
  Dcl_U/1 -> [U_DC_Link]
  [U_DC_Link] -> HV-DcDc_Converter_Master/4
  [U_DC_Link] -> HV-DcDc_Converter_Slave1/4
  [U_DC_Link] -> HV-DcDc_Converter_Slave/4(Dcl_U)
  [U_DC_Link] -> HV-DcDc_Converter_Slave3/4
  [Pmax4] -> Pmax/4
  [Pmax2] -> Pmax/2
  [Pmax3] -> Pmax/3
  [Pmax5] -> Pmax/5
  [Pmax1] -> Pmax/1
  Pdc/1 -> Terminator/1
  HV-DcDc_Converter_Master/1 -> [P_bat1]
  [P_bat1] -> P_bat/1
  Determine Hdc_P_max_vec/1(Hdc_P_max_vec) -> Bus Creator/3  "Hdc_P_max_vec"
  [Emg_P_dcDemand_Bat1] -> HV-DcDc_Converter_Master/3
  [Emg_P_dcDemand_Bat3] -> HV-DcDc_Converter_Slave1/3
  [Emg_P_dcDemand_Bat4] -> HV-DcDc_Converter_Slave2/3
  [Emg_P_dcDemand_Bat5] -> HV-DcDc_Converter_Slave3/3
  [Hvb_U_Bat1] -> HV-DcDc_Converter_Master/1
  [Hvb_U_Bat2] -> HV-DcDc_Converter_Slave/1(Hvb_U_Bat)
  [Hvb_U_Bat4] -> HV-DcDc_Converter_Slave2/1
  [Hvb_U_Bat5] -> HV-DcDc_Converter_Slave3/1
  [Hvb_U_Bat3] -> HV-DcDc_Converter_Slave1/1
  Bus Selector/3 -> HV-DcDc_Converter_Slave/5(case)  "<signal12>"
  Dcl_P_total/1 -> ?
  [Emg_P_dcDemand_Bat2] -> HV-DcDc_Converter_Slave/3(Emg_P_dcDemand)

== system HVModAL_Fahrzeugmodell/Sim_Control ==
  1-D Lookup Table : Lookup_n-D  NumberOfTableDimensions=1  BreakpointsForDimension1=[0.1 0.2 0.5 1 2 3]  Table=[1 0.98 0.93 0.85 0.72 0.62]  InternalRulePriority=Speed  RndMeth=Simplest  InputSameDT=on
  Bus Selector : BusSelector  OutputSignals=SB_Bat1,SB_Bat2
  Bus Selector1 : BusSelector  OutputSignals=V_Stackvoltage_V,P_max_discharge_10s_W
  Bus Selector2 : BusSelector  OutputSignals=V_Stackvoltage_V,P_max_discharge_10s_W,single_battery
  Bus Selector3 : BusSelector  OutputSignals=signal13
  Clock : Clock
  Compare To Constant : simulink/Logic and Bit Operations/Compare To Constant  relop=<=  const=100  OutDataTypeStr=boolean
  Compare To Constant1 : simulink/Logic and Bit Operations/Compare To Constant  relop=<=  const=100  OutDataTypeStr=boolean
  Compare To Constant2 : simulink/Logic and Bit Operations/Compare To Constant  relop=>  const=10  OutDataTypeStr=boolean
  Compare To Constant3 : simulink/Logic and Bit Operations/Compare To Constant  relop=<  const=0  OutDataTypeStr=boolean
  Compare To Constant4 : simulink/Logic and Bit Operations/Compare To Constant  relop=<  const=0  OutDataTypeStr=boolean
  Compare To Constant5 : simulink/Logic and Bit Operations/Compare To Constant  relop=>=  const=100  OutDataTypeStr=boolean
  Constant : Constant  Value=3
  Integrator : Integrator
  Logical Operator : Logic  Inputs=3  AllPortsSameDT=off  OutDataTypeStr=boolean
  Logical Operator1 : Logic  AllPortsSameDT=off  OutDataTypeStr=boolean
  Logical Operator2 : Logic  Operator=OR  Inputs=5  AllPortsSameDT=off  OutDataTypeStr=boolean
  Logical Operator3 : Logic  AllPortsSameDT=off  OutDataTypeStr=boolean
  Product : Product
  Relational Operator4 : RelationalOperator  Operator=>  OutDataTypeStr=boolean
  Scope{,1..2,4..5} (5 alike) : Scope
  Speed : Subsystem
  Stop Simulation : Stop
  tag scope: SimCtrl_ToLogging=global
  wires:
  Logical Operator3/1 -> Logical Operator2/1
  Logical Operator/1 -> Logical Operator2/3
  Logical Operator1/1 -> Logical Operator2/2
  Logical Operator2/1 -> Stop Simulation/1, [SimCtrl_ToLogging]
  Compare To Constant4/1 -> Logical Operator1/2
  Compare To Constant3/1 -> Logical Operator3/1
  Bus Selector2/1 -> Compare To Constant4/1  "<V_Stackvoltage_V>"
  Bus Selector1/1 -> Compare To Constant3/1  "<V_Stackvoltage_V>"
  Compare To Constant2/1 -> Logical Operator/3, Logical Operator1/1, Logical Operator3/2
  Clock/1 -> Compare To Constant2/1
  Compare To Constant1/1 -> Logical Operator/2
  Compare To Constant/1 -> Logical Operator/1
  Bus Selector2/2 -> Integrator/1, Compare To Constant1/1  "<P_max_discharge_10s_W>"
  Bus Selector1/2 -> Compare To Constant/1  "<P_max_discharge_10s_W>"
  Bus Selector/2 -> Bus Selector2/1  "<SB_Bat2>"
  Bus Selector/1 -> Bus Selector1/1  "<SB_Bat1>"
  [Hvb_SWbus_toworkspace] -> Bus Selector/1
  Speed/3(v_deviation(km/h)) -> Compare To Constant5/1  "v_deviation(km/h)"
  Speed/1(v_cycle(km/h)) -> ?  "v_cycle(km/h)"
  Speed/2(v_actual(km/h)) -> ?  "v_actual(km/h)"
  Compare To Constant5/1 -> Logical Operator2/4
  Bus Selector2/3 -> Product/1  "<single_battery>"
  1-D Lookup Table/1 -> Scope4/1, Product/2
  [EMG_BusSW_ToWorkspace] -> Bus Selector3/1
  Product/1 -> Scope/1, Relational Operator4/2
  Integrator/1 -> Scope2/1, Relational Operator4/1
  Relational Operator4/1 -> Scope1/1
  Constant/1 -> 1-D Lookup Table/1

== system HVModAL_Fahrzeugmodell/To Workspace (Two) ==
  note: Warning:
      | one signal in veh disconnected
      | When connected: port width problems
  Aux : Subsystem
  Bus Creator1 : BusCreator  Inputs=10
  Clock : Clock
      settings: Decimation=100
  Data Logging : Subsystem  TreatAsAtomicUnit=on
  Dcl : Subsystem
  Debug Mode on/off : Constant  Value=sim_params.debug_mode
  Drp : Subsystem
  Elm : Subsystem
  Emg : Subsystem
  Hdc : Subsystem
  Hvb : Subsystem
  Tri : Subsystem
  Veh : Subsystem
  wires:
  Debug Mode on/off/1 -> Data Logging/Enable
  Bus Creator1/1 -> Data Logging/1(result_Bus)  "result_Bus"
  Dcl/1(Dcl bus) -> Bus Creator1/5  "Dcl"
  Hdc/1(Hdc bus) -> Bus Creator1/6  "Hdc"
  Elm/1(Elm bus) -> Bus Creator1/4  "Elm"
  Veh/1(Veh bus) -> Bus Creator1/2  "Veh"
  Clock/1 -> Bus Creator1/10  "clock"
  Tri/1(Tri bus) -> Bus Creator1/3  "Tri"
  Drp/1(Drp bus) -> Bus Creator1/7  "Drp"
  Hvb/1(Hvb_PB) -> Bus Creator1/1  "Hvb"
  Emg/1(Drp bus) -> Bus Creator1/8  "Emg"
  Aux/1(Aux_bus) -> Bus Creator1/9  "Aux"

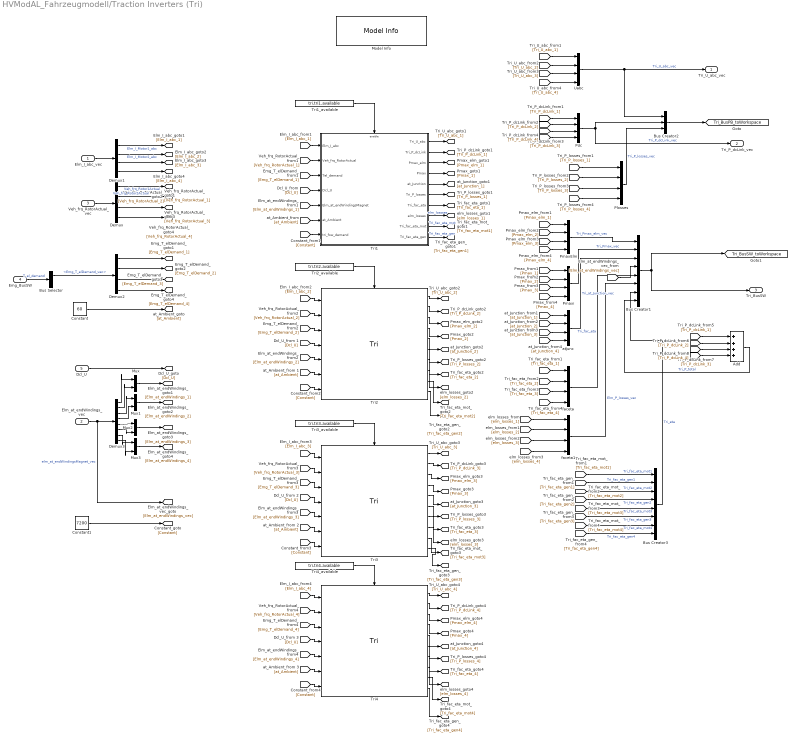
== system HVModAL_Fahrzeugmodell/Traction Inverters (Tri) ==
  Elm_I_abc_vec : Inport
  Elm_at_endWindings_vec : Inport  Port=2
  Veh_frq_RotorActual_vec : Inport  Port=3
  Emg_BusSW : Inport  Port=4
  Dcl_U : Inport  Port=5
  Add : Sum  Inputs=++++
  Bus Creator1 : BusCreator  Inputs=8
  Bus Creator2 : BusCreator  Inputs=3
  Bus Creator3 : BusCreator  Inputs=8
  Bus Selector : BusSelector  OutputSignals=Emg_T_elDemand_vec,Emg_at_Ambient
  Constant : Constant  Value=60
  Constant1 : Constant  Value=7200
  Demux : Demux
  Demux1 : Demux
  Demux2 : Demux
  Demux3 : Demux  Outputs=8
  Model Info : simulink/Model-Wide Utilities/Model Info  Frame=on  DisplayStringWithTags=|  HorizontalTextAlignment=Center  LeftAlignmentValue=0.5  SourceBlockDiagram=HVModAL_Fahrzeugmodell  TagMaxNumber=20
      | Responsibility
      | ISEA
      | 
      | Model Version: %<ModelVersion>
      | Last modified: %<LastModificationDate>
  Mux{,1..3} (4 alike) : Mux  Inputs=2
  Pdc : Mux
  Plosses : Mux
  PmaxElm : Mux
  "Pmaxi " : Mux
  Tri1 : Subsystem  AncestorBlock=lib_tri_modules/Tri  mask{TRIname=tri.tri1, ELMname=elm.elm1}
      mask prompts: TRIname "TRI Struct"; ELMname "ELM Struct"
  Tri1_available : Constant  Value=tri.tri1.available
  Tri2 : lib_tri_modules/Tri  TRIname=tri.tri2  ELMname=elm.elm2
  Tri2_available : Constant  Value=tri.tri2.available
  Tri3 : lib_tri_modules/Tri  TRIname=tri.tri3  ELMname=elm.elm3
  Tri3_available : Constant  Value=tri.tri3.available
  Tri4 : lib_tri_modules/Tri  TRIname=tri.tri4  ELMname=elm.elm4
  Tri4_available : Constant  Value=tri.tri4.available
  Uabc : Mux
  atJunc : Mux
  faceta : Mux
  faceta1 : Mux
  Tri_U_abc_vec : Outport
  Tri_P_dcLink_vec : Outport  Port=2
  "Tri_BusSW " : Outport  Port=3
  tag scope: Tri_BusPB_toWorkspace=global, Tri_BusSW_toWorkspace=global
  wires:
  Emg_BusSW/1 -> Bus Selector/1  "T_el_demand"
  Veh_frq_RotorActual_vec/1 -> Demux/1
  Elm_I_abc_vec/1 -> Demux1/1
  Bus Selector/1 -> Demux2/1  "<Emg_T_elDemand_vec>"
  Tri1/1(Tri_U_abc) -> [Tri_U_abc_1]
  Tri1_available/1 -> Tri1/Enable
  "Pmaxi "/1 -> Bus Creator1/2  "Tri_Pmax_vec"
  PmaxElm/1 -> Bus Creator1/1  "Tri_Pmax_elm_vec"
  atJunc/1 -> Bus Creator1/3  "Tri_at_Junction_vec"
  Bus Creator1/1 -> "Tri_BusSW "/1, [Tri_BusSW_toWorkspace]
  Tri2_available/1 -> Tri2/Enable
  Bus Creator2/1 -> [Tri_BusPB_toWorkspace]
  Pdc/1 -> Tri_P_dcLink_vec/1, Bus Creator2/2  "Tri_P_dcLink_vec"
  Uabc/1 -> Bus Creator2/1, Tri_U_abc_vec/1  "Tri_U_abc_vec"
  Plosses/1 -> Bus Creator2/3  "Tri_P_losses_vec"
  Tri3_available/1 -> Tri3/Enable
  Dcl_U/1 -> [Dcl_U]
  faceta/1 -> Bus Creator1/5  "Tri_fac_eta"
  Constant1/1 -> [Constant]
  Demux1/1 -> [Elm_I_abc_1]  "Elm_I_Motor1_abc"
  [Elm_I_abc_1] -> Tri1/1(Elm_I_abc)
  Demux/1 -> [Veh_frq_RotorActual_1]  "Veh_frq_Rotor1Actual"
  [Veh_frq_RotorActual_1] -> Tri1/2(Veh_frq_RotorActual)
  Demux2/1 -> [Emg_T_elDemand_1]
  [Emg_T_elDemand_1] -> Tri1/3(Tel_demand)
  [at_Ambient] -> Tri1/6(at_Ambient)
  Elm_at_endWindings_vec/1 -> Demux3/1, [Elm_at_endWindings_vec]  "elm_at_endWindingsMagnet_vec"
  [Dcl_U] -> Tri1/4(Dcl_U)
  [Elm_at_endWindings_1] -> Tri1/5(Elm_at_endWindingsMagnet)
  [Constant] -> Tri1/7(tri_fsw_demand)
  Demux1/2 -> [Elm_I_abc_2]  "Elm_I_Motor2_abc"
  [Elm_I_abc_2] -> Tri2/1
  Demux/2 -> [Veh_frq_RotorActual_2]  "Veh_frq_Rotor2Actual"
  [Veh_frq_RotorActual_2] -> Tri2/2
  Demux2/2 -> [Emg_T_elDemand_2]
  [Emg_T_elDemand_2] -> Tri2/3
  [Dcl_U] -> Tri2/4
  [Elm_at_endWindings_2] -> Tri2/5
  [Constant] -> Tri2/7
  [at_Ambient] -> Tri2/6
  Demux1/3 -> [Elm_I_abc_3]
  [Elm_I_abc_3] -> Tri3/1
  Demux/3 -> [Veh_frq_RotorActual_3]
  [Veh_frq_RotorActual_3] -> Tri3/2
  Demux2/3 -> [Emg_T_elDemand_3]
  [Emg_T_elDemand_3] -> Tri3/3
  [Dcl_U] -> Tri3/4
  [Elm_at_endWindings_3] -> Tri3/5
  [at_Ambient] -> Tri3/6
  Tri4_available/1 -> Tri4/Enable
  Demux1/4 -> [Elm_I_abc_4]
  Demux/4 -> [Veh_frq_RotorActual_4]
  Demux2/4 -> [Emg_T_elDemand_4]
  [Elm_I_abc_4] -> Tri4/1
  [Veh_frq_RotorActual_4] -> Tri4/2
  [Emg_T_elDemand_4] -> Tri4/3
  [Dcl_U] -> Tri4/4
  [Elm_at_endWindings_4] -> Tri4/5
  [at_Ambient] -> Tri4/6
  [Elm_at_endWindings_vec] -> Bus Creator1/4
  [Tri_U_abc_1] -> Uabc/1
  Tri2/1 -> [Tri_U_abc_2]
  [Tri_U_abc_2] -> Uabc/2
  Tri3/1 -> [Tri_U_abc_3]
  [Tri_U_abc_3] -> Uabc/3
  Tri4/1 -> [Tri_U_abc_4]
  [Tri_U_abc_4] -> Uabc/4
  [Tri_P_dcLink_1] -> Pdc/1
  Tri1/2(Tri_P_dcLink) -> [Tri_P_dcLink_1]
  Tri2/2 -> [Tri_P_dcLink_2]
  [Tri_P_dcLink_2] -> Pdc/2
  Tri3/2 -> [Tri_P_dcLink_3]
  Tri4/2 -> [Tri_P_dcLink_4]
  [Tri_P_dcLink_3] -> Pdc/3
  [Tri_P_dcLink_4] -> Pdc/4
  [Pmax_elm_1] -> PmaxElm/1
  Tri1/3(Pmax_elm) -> [Pmax_elm_1]
  Tri2/3 -> [Pmax_elm_2]
  [Pmax_elm_2] -> PmaxElm/2
  [Pmax_elm_3] -> PmaxElm/3
  Tri3/3 -> [Pmax_elm_3]
  Tri4/3 -> [Pmax_elm_4]
  [Pmax_elm_4] -> PmaxElm/4
  Tri1/4(Pmax) -> [Pmax_1]
  [Pmax_1] -> "Pmaxi "/1
  Tri2/4 -> [Pmax_2]
  [Pmax_2] -> "Pmaxi "/2
  [Pmax_3] -> "Pmaxi "/3
  Tri3/4 -> [Pmax_3]
  Tri4/4 -> [Pmax_4]
  [Pmax_4] -> "Pmaxi "/4
  [at_Junction_1] -> atJunc/1
  Tri1/5(at_Junction) -> [at_Junction_1]
  Tri2/5 -> [at_Junction_2]
  [at_Junction_2] -> atJunc/2
  [at_Junction_3] -> atJunc/3
  Tri3/5 -> [at_Junction_3]
  Tri4/5 -> [at_Junction_4]
  [at_Junction_4] -> atJunc/4
  Tri1/6(Tri_P_losses) -> [Tri_P_losses_1]
  [Tri_P_losses_1] -> Plosses/1
  [Tri_P_losses_2] -> Plosses/2
  Tri2/6 -> [Tri_P_losses_2]
  Tri4/6 -> [Tri_P_losses_4]
  Tri3/6 -> [Tri_P_losses_3]
  [Tri_P_losses_3] -> Plosses/3
  [Tri_P_losses_4] -> Plosses/4
  Tri1/7(Tri_fac_eta) -> [Tri_fac_eta_1]
  [Tri_fac_eta_1] -> faceta/1
  Tri1/8(elm_losses) -> [elm_losses_1]  "elm_lossses"
  [elm_losses_1] -> faceta1/1
  faceta1/1 -> Bus Creator1/6  "Elm_P_losses_vec"
  [Constant] -> Tri3/7
  [Constant] -> Tri4/7
  Tri2/7 -> [Tri_fac_eta_2]
  Tri2/8 -> [elm_losses_2]
  [Tri_fac_eta_2] -> faceta/2
  [elm_losses_2] -> faceta1/2
  [Tri_fac_eta_3] -> faceta/3
  [Tri_fac_eta_4] -> faceta/4
  Tri3/7 -> [Tri_fac_eta_3]
  Tri3/8 -> [elm_losses_3]
  Tri4/7 -> [Tri_fac_eta_4]
  Tri4/8 -> [elm_losses_4]
  [elm_losses_3] -> faceta1/3
  [elm_losses_4] -> faceta1/4
  Demux3/1 -> Mux/1
  Demux3/2 -> Mux/2
  Mux/1 -> [Elm_at_endWindings_1]
  Demux3/3 -> Mux1/1
  Demux3/4 -> Mux1/2
  Mux1/1 -> [Elm_at_endWindings_2]
  Demux3/5 -> Mux2/1
  Demux3/6 -> Mux2/2
  Mux2/1 -> [Elm_at_endWindings_3]
  Demux3/7 -> Mux3/1
  Demux3/8 -> Mux3/2
  Mux3/1 -> [Elm_at_endWindings_4]
  Tri2/9 -> [Tri_fac_eta_mot2]
  [Tri_fac_eta_mot2] -> Bus Creator3/3  "Tri_fac_eta_mot2"
  Tri4/9 -> [Tri_fac_eta_mot4]
  Bus Creator3/1 -> Bus Creator1/7  "Tri_eta"
  Tri2/10 -> [Tri_fac_eta_gen2]
  [Tri_fac_eta_gen2] -> Bus Creator3/4  "Tri_fac_eta_gen2"
  Tri1/9(Tri_fac_eta_mot) -> [Tri_fac_eta_mot1]  "Tri_fac_eta_mot"
  Tri1/10(Tri_fac_eta_gen) -> [Tri_fac_eta_gen1]  "Tri_fac_eta_gen"
  [Tri_fac_eta_gen1] -> Bus Creator3/2  "Tri_fac_eta_gen1"
  [Tri_fac_eta_mot1] -> Bus Creator3/1  "Tri_fac_eta_mot1"
  Tri3/9 -> [Tri_fac_eta_mot3]
  Tri3/10 -> [Tri_fac_eta_gen3]
  [Tri_fac_eta_mot3] -> Bus Creator3/5  "Tri_fac_eta_mot3"
  [Tri_fac_eta_gen3] -> Bus Creator3/6  "Tri_fac_eta_gen3"
  Tri4/10 -> [Tri_fac_eta_gen4]
  [Tri_fac_eta_mot4] -> Bus Creator3/7  "Tri_fac_eta_mot4"
  [Tri_fac_eta_gen4] -> Bus Creator3/8  "Tri_fac_eta_gen4"
  Constant/1 -> [at_Ambient]
  [Tri_P_dcLink_1] -> Add/1
  [Tri_P_dcLink_2] -> Add/2
  [Tri_P_dcLink_4] -> Add/4
  [Tri_P_dcLink_3] -> Add/3
  Add/1 -> Bus Creator1/8  "Tri_P_total"

== system HVModAL_Fahrzeugmodell/Vehicle_Chassis (Veh) ==
  note: Addition of electrical and
      | mechanical torque
  note: Mechanical brake
  Elm_T_el_vec : Inport
  Drp_rad_RoadSlope : Inport  Port=2
  Emg_BusSW : Inport  Port=3
  1/r_dyn : Gain  Gain=1/veh.wheel.radius  SaturateOnIntegerOverflow=on  OutDataTypeStr=Inherit: Same as input  ParamDataTypeStr=Inherit: Same as input
  Add : Sum
  Axle Load : Subsystem
  Bus Creator : BusCreator  Inputs=8
  Bus Selector : BusSelector  OutputSignals=Emg_T_mechDemand,Emg_Gearbox_vec
  Bus Selector1 : BusSelector  OutputSignals=gearboxratio_vec,Gear change
  Calculate Reduced Vehicle Mass : Subsystem
  Constant : Constant
  Delay : Delay  DelayLength=1  InitialCondition=0
  Delay1 : Delay  DelayLength=1  SampleTime=sim_params.Ts
  Delay2 : Delay  DelayLength=1  InitialCondition=0
  Delay3 : Delay  DelayLength=1  InitialCondition=0
  Demux : Demux
  Demux1 : Demux
  Demux2 : Demux
  Drive Shaft : Subsystem
  Driving Data : Subsystem
  Driving Forces : Subsystem
  Gearbox1 : lib_gearbox/Gearbox  mask{gearbox=veh.gearbox.gearbox1}
      mask prompts: gearbox "Gearbox Struct"
  Gearbox2 : lib_gearbox/Gearbox  mask{gearbox=veh.gearbox.gearbox2}
      mask prompts: gearbox "Gearbox Struc"
  Gearbox3 : lib_gearbox/Gearbox  mask{gearbox=veh.gearbox.gearbox3}
      mask prompts: gearbox "Gearbox Struct"
  Gearbox4 : lib_gearbox/Gearbox  mask{gearbox=veh.gearbox.gearbox4}
      mask prompts: gearbox "Gearbox Struct"
  Interruption of Traction / Clutch : Subsystem
  Max Driving Force : Subsystem
  Model Info : simulink/Model-Wide Utilities/Model Info  Frame=on  DisplayStringWithTags=|  HorizontalTextAlignment=Center  LeftAlignmentValue=0.5  SourceBlockDiagram=HVModAL_Fahrzeugmodell  TagMaxNumber=20
      | Responisbility
      | Bosch
      | 
      | Model Version: %<ModelVersion>
      | Last modified: %<LastModificationDate>
  Mux : Mux  Inputs=5
  Mux1 : Mux
  Wheel Model : Subsystem
  Wheelload : Subsystem
  rpm->frq : Gain  Gain=1/60  SaturateOnIntegerOverflow=on  OutDataTypeStr=Inherit: Same as input  ParamDataTypeStr=Inherit: Same as input
  Veh_BusSW : Outport
  Veh_frq_machineRotor_vec : Outport  Port=2
  tag scope: Veh_SWBus_toworkspace=global
  wires:
  Driving Data/2(v_wheel(m/s)) -> Wheel Model/2(v_wheel[m/s]), Delay1/1, Bus Creator/3  "Veh_v_wheel"
  rpm->frq/1 -> Bus Creator/1, Veh_frq_machineRotor_vec/1  "Veh_frq_machineRotor_vec"
  Bus Creator/1 -> Veh_BusSW/1, [Veh_SWBus_toworkspace]
  Constant/1 -> Bus Creator/2  "Veh_random"
  Emg_BusSW/1 -> Bus Selector/1
  Bus Selector/1 -> 1/r_dyn/1  "<Emg_T_mechDemand>"
  1/r_dyn/1 -> Add/2  "F_brake(N)"
  Driving Data/3(a_actual [m/s]) -> Bus Creator/4, Delay3/1, Wheel Model/1(a_actual [m/s^2])  "Veh_a_actual"
  Demux/2 -> Gearbox2/1
  Driving Data/1(n_motor(rpm)) -> Demux1/1, rpm->frq/1
  Demux1/1 -> Gearbox1/2
  Demux1/2 -> Gearbox2/2
  Demux1/3 -> Gearbox3/2
  Drive Shaft/1(F_acc(N)) -> Add/1
  Demux/3 -> Gearbox3/1
  Demux/1 -> Gearbox1/1
  Elm_T_el_vec/1 -> Demux/1
  Wheel Model/1(v_actual[m/s]) -> Bus Creator/6  "Veh_v_actual"
  Axle Load/2(back_load [N]) -> Wheelload/2(Back_load [N]), Max Driving Force/2(back_load [N])
  Max Driving Force/1(T_wheels_max) -> Bus Creator/5  "T_wheels_max_vec"
  Wheelload/1(Wheelload [N]) -> Wheel Model/4(WheelLoad [N])
  Add/1 -> Delay/1
  Drp_rad_RoadSlope/1 -> Delay2/1
  Delay2/1 -> Driving Forces/2(grad_cycle(rad)), Axle Load/2(grad_cycle (rad))
  Delay1/1 -> Driving Forces/3(v_actual(m/s))  "Veh_v_actual"
  Driving Forces/2(F_aero) -> Mux/2
  Driving Forces/5(F_acc) -> Mux/1
  Driving Forces/4(F_climb) -> Mux/3
  Driving Forces/1(F_drive(N)) -> Driving Data/2(F_drive [N]), Wheel Model/3(F_wheel [N]), Mux/4
  Driving Forces/3(F_roll) -> Mux/5
  Mux/1 -> Bus Creator/7  "Veh_DrivingForces_N"
  Gearbox1/1 -> Mux1/1
  Mux1/1 -> Bus Creator/8  "Veh_Ploss_gearbox_vec"
  Gearbox1/2 -> Drive Shaft/1(Tin1)
  Gearbox2/2 -> Drive Shaft/2(Tin2)
  Gearbox3/2 -> Drive Shaft/3(Tin3)
  Gearbox4/2 -> Drive Shaft/4(Tin4)
  Gearbox2/1 -> Mux1/2
  Gearbox3/1 -> Mux1/3
  Gearbox4/1 -> Mux1/4
  Axle Load/1(front_load [N]) -> Wheelload/1(Front_load [N]), Max Driving Force/1(front_load [N])
  Calculate Reduced Vehicle Mass/1(m_red(kg)) -> Driving Data/1(m_red [kg])
  Demux1/4 -> Gearbox4/2
  Demux/4 -> Gearbox4/1
  Bus Selector1/1 -> Demux2/1  "<gearboxratio_vec>"
  Delay/1 -> Interruption of Traction / Clutch/1(F_acc[N])
  Bus Selector1/2 -> Interruption of Traction / Clutch/2(Gearchange)  "<Gear change>"
  Interruption of Traction / Clutch/1(F_acc_actual[N]) -> Driving Forces/1(F_acc(N))
  Bus Selector/2 -> Bus Selector1/1, [gearboxratio]  "<Emg_Gearbox_vec>"
  [gearboxratio] -> Driving Data/3(Emg_gearbox_vec)
  Delay3/1 -> Axle Load/1(a_actual (m/s^2))
  Demux2/4 -> Gearbox4/3
  Demux2/3 -> Gearbox3/3
  Demux2/2 -> Gearbox2/3
  Demux2/1 -> Gearbox1/3
